simulink model "Main_Simulink"  (R2023b)
settings: Solver=FixedStepDiscrete  StartTime=0.0  StopTime=inf  FixedStep=0.001  RelTol=1e-3
undefined symbols (not defined in the file or in its folder): battery_builder_rtmsupport, gcbh, Initial_SOC
libraries: nesl_utility x118, pack_105s34p_structured_lib x105, fl_lib x14, ee_lib x7, dspstat3 x6, BatteryBalancing x1, deeplib x1
(part 3 of 10)

== system Main_Simulink/Battery Management System/State of Power Estimation System/Maximum Charge Power Limits/For Each Subsystem1 ==
  Temp : Inport  Partition=on  PartitionDimension=1  PartitionWidth=1  PartitionOffset=0
  HVBatSOCMin : Inport  Port=2
  For Each : ForEach  DisableCoverage=on
  Pack Charge Power Limit - 10s : Lookup_n-D  BreakpointsForDimension1=[-30;-20;-10;0;10;20;30;40;50;60]  BreakpointsForDimension2=[0 5 10 15 20 25 30 35 40 45 50 55 60 65 70 75 80 85 90 95 100]  Table=[0 0 0 0 0 0 0 0 0 0 0 0 0 0 0 0 0 0 0 0 0;0 0 0 0 0 0 0 0 0 0 0 0 0 0 0 0 0 0 0 0 0;19.76749 19.76749 19.65082 20.01926 20.36403 19.91161 19.53766 17.74126 15.90855 13.98243 12.04796 10.11331 8.150748 6.165785 4.146483 4.194749 4.24254 2.863269 1.449165 0.729806 0;37.15349 37.25908 37.36467 37.99491 38.68739 37.01292 35.57943 34.03129 32.33249 28.38431 24.39997 22.5555 20.67389 16.66823 12.60507 10.58905 8.539529 6.477517 4.366351 2.192535 0;50.75138 51.59179 51.65872 52.84392 54.27789 52.74104 51.43037 49.99522 48.55512 44.79444 41.00328 35.11689 29.12726 25.2468 21.25129 17.16492 12.9983 10.91332 8.795933 4.432558 0;67.50776 69.05614 69.22503 70.87652 72.7677 72.79337 73.0761 69.11144 65.03528 61.39678 57.74562 50.54301 43.23853 38.08701 32.7453 27.30376 21.75319 18.2489 14.69784 7.398185 0;75.51099 77.37549 77.95205 79.80169 81.84837 82.63384 83.74967 78.51018 73.16383 69.64374 66.0563 58.24337 50.28199 44.49695 38.47487 32.35472 26.12019 21.90894 17.64118 8.874131 0;74.46151 76.49357 77.35464 79.22241 81.36253 82.08661 83.22665 78.09122 72.77178 69.28399 65.77915 57.99753 50.09838 44.31755 38.34415 32.22712 26.01267 21.84759 17.61682 8.847446 0;48.00354 49.35825 50.19251 51.64039 53.2093 53.79276 54.56109 51.26258 47.84552 45.59639 43.32059 38.26118 33.1039 29.30947 25.39243 21.36695 17.26419 14.51359 11.71338 5.890391 0;0 0 0 0 0 0 0 0 0 0 0 0 0 0 0 0 0 0 0 0 0]  InternalRulePriority=Speed  RndMeth=Simplest
      settings: InputPortMap=u0,u1
  Out1 : Outport  ConcatenationDimension=1
  wires:
  HVBatSOCMin/1 -> Pack Charge Power Limit - 10s/2
  Temp/1 -> Pack Charge Power Limit - 10s/1
  Pack Charge Power Limit - 10s/1 -> Out1/1

== system Main_Simulink/Battery Management System/State of Power Estimation System/Maximum Charge Power Limits/For Each Subsystem2 ==
  Temp : Inport  Partition=on  PartitionDimension=1  PartitionWidth=1  PartitionOffset=0
  HVBatSOCMin : Inport  Port=2
  For Each : ForEach  DisableCoverage=on
  Pack Charge Power Limit - 2s : Lookup_n-D  BreakpointsForDimension1=[-30;-20;-10;0;10;20;30;40;50;60]  BreakpointsForDimension2=[0 5 10 15 20 25 30 35 40 45 50 55 60 65 70 75 80 85 90 95 100]  Table=[0 0 0 0 0 0 0 0 0 0 0 0 0 0 0 0 0 0 0 0 0;0 0 0 0 0 0 0 0 0 0 0 0 0 0 0 0 0 0 0 0 0;19.58352 19.58352 19.45651 19.84169 20.21864 19.8213 19.46671 17.67557 15.85694 13.94558 12.01771 10.09422 8.137316 6.159089 4.143376 4.191016 4.238837 2.861684 1.448811 0.72974 0;36.49456 36.60015 36.70574 37.48533 38.32484 36.81065 35.41273 33.83658 32.2081 28.27762 24.32648 22.49047 20.61798 16.63012 12.57878 10.57114 8.529705 6.471868 4.364553 2.192111 0;49.59029 50.43071 50.70087 52.14778 53.75303 52.35297 51.03415 49.65909 48.22489 44.53214 40.77991 34.95857 29.0243 25.154 21.18801 17.12293 12.9785 10.89967 8.788762 4.430448 0;65.59661 67.14499 67.90263 69.84698 72.06978 72.21885 72.5005 68.58984 64.57818 61.01484 57.37573 50.30478 43.06975 37.92462 32.63123 27.2283 21.70777 18.22059 14.68121 7.393929 0;73.18842 75.05293 76.34885 78.58837 81.05583 82.06849 83.18148 77.97854 72.71563 69.2522 65.72517 57.97825 50.09367 44.30032 38.34697 32.26844 26.06097 21.87292 17.6235 8.869533 0;71.97071 74.00277 75.69889 78.01635 80.51607 81.53568 82.69007 77.60201 72.42077 68.96612 65.46512 57.75822 49.92863 44.16534 38.24005 32.15085 25.96253 21.81627 17.60159 8.843684 0;46.89652 48.25122 49.45662 51.10436 52.8331 53.5479 54.32261 51.04516 47.68952 45.45511 43.18102 38.15483 33.02845 29.24182 25.34616 21.33306 17.24191 14.49967 11.70661 5.888719 0;0 0 0 0 0 0 0 0 0 0 0 0 0 0 0 0 0 0 0 0 0]  InternalRulePriority=Speed  RndMeth=Simplest
      settings: InputPortMap=u0,u1
  Out1 : Outport  ConcatenationDimension=1
  wires:
  HVBatSOCMin/1 -> Pack Charge Power Limit - 2s/2
  Temp/1 -> Pack Charge Power Limit - 2s/1
  Pack Charge Power Limit - 2s/1 -> Out1/1

== system Main_Simulink/Battery Management System/State of Power Estimation System/Maximum Charge Power Limits/For Each Subsystem3 ==
  Temp : Inport  Partition=on  PartitionDimension=1  PartitionWidth=1  PartitionOffset=0
  HVBatSOCMin : Inport  Port=2
  For Each : ForEach  DisableCoverage=on
  Pack Charge Power Limit - 30s : Lookup_n-D  BreakpointsForDimension1=[-30;-20;-10;0;10;20;30;40;50;60]  BreakpointsForDimension2=[0 5 10 15 20 25 30 35 40 45 50 55 60 65 70 75 80 85 90 95 100]  Table=[0 0 0 0 0 0 0 0 0 0 0 0 0 0 0 0 0 0 0 0 0;0 0 0 0 0 0 0 0 0 0 0 0 0 0 0 0 0 0 0 0 0;0 0 0 0 0 0 0 0 0 0 0 0 0 0 0 0 0 0 0 0 0;8.039485 8.064123 8.088761 8.279835 8.501733 8.660965 8.837547 8.974482 9.110076 7.866004 6.603531 6.683109 6.761689 5.473014 4.152702 4.200954 4.248799 2.866871 1.450526 0.729607 0;11.3011 11.5012 11.63529 12.01056 12.40712 12.57062 12.75608 12.93391 13.1115 13.24873 13.3883 13.56159 13.73198 13.9362 14.11972 13.57803 13.02453 10.92908 8.805357 4.435029 0;14.96331 15.33197 15.57367 16.06785 16.58759 16.79556 17.03852 17.27949 17.51753 17.70142 17.88948 18.11963 18.34425 18.62175 18.85959 18.86453 18.86253 15.32536 11.7483 5.916568 0;20.71779 21.26037 21.60042 22.24946 22.91092 23.18255 23.52677 23.84754 24.16825 24.42631 24.69339 25.006 25.31353 24.50762 23.60729 22.69796 21.75837 17.50956 13.21299 6.651374 0;28.3715 29.17787 29.59744 30.45927 31.35956 31.68052 32.17173 32.61593 33.0527 33.41197 33.7704 34.18493 34.60144 31.54245 28.32199 25.02635 21.66624 17.46263 13.19626 6.631388 0;16.60354 17.08736 17.43194 18.00695 18.5958 18.82348 19.11245 19.38268 19.65023 19.86546 20.08039 20.33233 20.58498 20.88514 21.15023 17.79983 14.38194 13.06513 11.72123 5.892346 0;0 0 0 0 0 0 0 0 0 0 0 0 0 0 0 0 0 0 0 0 0]  InternalRulePriority=Speed  RndMeth=Simplest
      settings: InputPortMap=u0,u1
  Out1 : Outport  ConcatenationDimension=1
  wires:
  HVBatSOCMin/1 -> Pack Charge Power Limit - 30s/2
  Temp/1 -> Pack Charge Power Limit - 30s/1
  Pack Charge Power Limit - 30s/1 -> Out1/1

== system Main_Simulink/Battery Management System/State of Power Estimation System/Maximum Charge Power Limits/For Each Subsystem4 ==
  Temp : Inport  Partition=on  PartitionDimension=1  PartitionWidth=1  PartitionOffset=0
  HVBatSOCMin : Inport  Port=2
  For Each : ForEach  DisableCoverage=on
  Pack Charge Power Limit - 180s : Lookup_n-D  BreakpointsForDimension1=[-30;-20;-10;0;10;20;30;40;50;60]  BreakpointsForDimension2=[0 5 10 15 20 25 30 35 40 45 50 55 60 65 70 75 80 85 90 95 100]  Table=[0 0 0 0 0 0 0 0 0 0 0 0 0 0 0 0 0 0 0 0 0;0 0 0 0 0 0 0 0 0 0 0 0 0 0 0 0 0 0 0 0 0;0 0 0 0 0 0 0 0 0 0 0 0 0 0 0 0 0 0 0 0 0;8.200519 8.225157 8.249795 8.449791 8.628751 8.713708 8.900788 9.041006 9.17303 7.90902 6.631868 6.710427 6.788544 5.492872 4.164691 4.209532 4.257341 2.870725 1.451275 0.729786 0;11.73069 11.93079 11.98528 12.24386 12.50444 12.65479 12.85775 13.02347 13.18717 13.32159 13.46314 13.63484 13.8141 14.0262 14.18781 13.64706 13.09032 10.96258 8.823694 4.44097 0;15.75103 16.11969 16.16875 16.4414 16.72958 16.92433 17.19946 17.41833 17.62262 17.80263 17.99554 18.22015 18.4672 18.74861 18.95158 18.96809 18.96715 15.37262 11.77152 5.926242 0;22.12594 22.66852 22.66387 22.907 23.15513 23.4058 23.7974 24.09552 24.35036 24.60225 24.8676 25.17956 25.53041 24.68474 23.72629 22.82709 21.87994 17.56221 13.23562 6.661459 0;31.06494 31.87131 31.6124 31.82007 31.86082 32.06269 32.65549 33.0561 33.38556 33.68284 34.05866 34.47747 34.96167 31.81577 28.4752 25.16758 21.7805 17.51312 13.21427 6.63946 0;17.57318 18.057 18.15732 18.49684 18.77626 18.96106 19.2866 19.54114 19.77006 19.96297 20.18416 20.43764 20.71466 21.00661 21.23642 17.87188 14.43273 13.09353 11.73546 5.898724 0;0 0 0 0 0 0 0 0 0 0 0 0 0 0 0 0 0 0 0 0 0]  InternalRulePriority=Speed  RndMeth=Simplest
      settings: InputPortMap=u0,u1
  Out1 : Outport  ConcatenationDimension=1
  wires:
  HVBatSOCMin/1 -> Pack Charge Power Limit - 180s/2
  Temp/1 -> Pack Charge Power Limit - 180s/1
  Pack Charge Power Limit - 180s/1 -> Out1/1

== system Main_Simulink/Battery Management System/State of Power Estimation System/Maximum Discharge Power Limits/For Each Subsystem ==
  Temp : Inport  Partition=on  PartitionDimension=1  PartitionWidth=1  PartitionOffset=0
  HVBatSOCMin : Inport  Port=2
  For Each : ForEach  DisableCoverage=on
  Pack Discharge Power Limit - 2s : Lookup_n-D  BreakpointsForDimension1=[-30;-20;-10;0;10;20;30;40;50;60]  BreakpointsForDimension2=[0 5 10 15 20 25 30 35 40 45 50 55 60 65 70 75 80 85 90 95 100]  Table=[0 0 0 0 0 0 0 0 0 0 0 0 0 0 0 0 0 0 0 0 0;0 1.6 3.2 6.9 10.5 10.9 11.4 11.6 11.8 12 12.2 18 23.6 24 24.4 24.8 25.1 25.5 25.9 26.4 26.8;0 2.8 5.4 8.4 11.5 22.7 33.8 34.4 35 35.5 35.9 41.8 47.8 48.5 49.2 49.9 50.5 51.4 52.3 58.6 65.1;0 5.4 10.7 21.7 33 39.3 45.5 46.4 47.2 53.2 59.1 59.9 60.8 67.2 73.8 74.7 75.6 76.8 78.1 78.7 79.6;0 10.9 21.9 33.9 46.6 53 59.5 66.1 73 73.8 74.6 81.6 88.7 90 91.2 98.6 106.4 113.2 120.4 121.6 122.7;0 16.2 32.8 50.5 69.1 75.8 82.6 89.5 96.7 97.8 98.9 106.2 113.5 115.2 116.7 124.5 132.3 139.8 147.3 148.9 150.4;0 16.3 33.1 97.7 160.7 163.9 166.7 169.9 172.6 175 177.1 179.7 182.2 185.1 187.7 190.3 192.9 195.2 197.2 199.5 201.3;0 16.2 33 97.8 162.1 164.9 168.1 170.8 173.9 176.1 178.2 180.7 183.2 185.7 188.4 191 194.5 196.2 198.7 200.6 202.2;0 10.9 22.2 34.3 47.2 53.8 60.5 67.3 74.3 75.2 76 83.2 90.5 91.7 93 94.2 95.6 103.1 110.9 111.9 112.8;0 0 0 0 0 0 0 0 0 0 0 0 0 0 0 0 0 0 0 0 0]  InternalRulePriority=Speed  RndMeth=Simplest
      settings: InputPortMap=u0,u1
  Out1 : Outport  ConcatenationDimension=1
  wires:
  HVBatSOCMin/1 -> Pack Discharge Power Limit - 2s/2
  Temp/1 -> Pack Discharge Power Limit - 2s/1
  Pack Discharge Power Limit - 2s/1 -> Out1/1

== system Main_Simulink/Battery Management System/State of Power Estimation System/Maximum Discharge Power Limits/For Each Subsystem1 ==
  Temp : Inport  Partition=on  PartitionDimension=1  PartitionWidth=1  PartitionOffset=0
  HVBatSOCMin : Inport  Port=2
  For Each : ForEach  DisableCoverage=on
  Pack Discharge Power Limit - 10s : Lookup_n-D  BreakpointsForDimension1=[-30;-20;-10;0;10;20;30;40;50;60]  BreakpointsForDimension2=[0 5 10 15 20 25 30 35 40 45 50 55 60 65 70 75 80 85 90 95 100]  Table=[0 0 0 0 0 0 0 0 0 0 0 0 0 0 0 0 0 0 0 0 0;0 1.6 3.2 6.8 10.4 10.9 11.3 11.6 11.8 12 12.1 17.9 23.4 23.8 24.2 24.6 24.9 25.3 25.8 26.2 26.6;0 2.7 5.4 8.3 11.4 22.6 33.5 34.2 34.8 35.2 35.6 41.4 47.2 48 48.7 49.4 50 50.8 51.7 57.9 64;0 5.4 10.6 21.4 32.7 39 45.2 46.1 47 52.9 58.7 59.5 60.2 66.6 73 73.8 74.6 75.8 77.1 78 78.7;0 10.8 21.7 33.6 46.1 52.5 58.9 65.4 72.1 73 73.8 80.6 87.6 88.8 90 97 104.3 111.3 118.4 119.7 120.3;0 16.1 32.4 50 68.4 75 81.7 83.1 84.5 91.1 97.8 105 112.1 113.6 115.1 122.5 130.1 137.7 145.1 146.8 147.6;0 16.2 32.8 61 90.2 97.2 104.2 111.2 118.5 125.4 132.3 139.7 147.2 154.9 162.3 170.2 178 186.2 194.3 196.5 197.2;0 16.1 32.7 61 90.4 97.4 104.5 111.8 119.1 126 133.1 140.3 148 155.4 163.2 171.2 179.5 187.6 196.5 198.3 198.8;0 10.8 22.1 34.1 46.9 53.5 60.2 67 73.9 74.7 75.6 82.6 89.9 91 92.3 93.5 94.8 102.4 110.3 111.2 111.8;0 0 0 0 0 0 0 0 0 0 0 0 0 0 0 0 0 0 0 0 0]  InternalRulePriority=Speed  RndMeth=Simplest
      settings: InputPortMap=u0,u1
  Out1 : Outport  ConcatenationDimension=1
  wires:
  HVBatSOCMin/1 -> Pack Discharge Power Limit - 10s/2
  Temp/1 -> Pack Discharge Power Limit - 10s/1
  Pack Discharge Power Limit - 10s/1 -> Out1/1

== system Main_Simulink/Battery Management System/State of Power Estimation System/Maximum Discharge Power Limits/For Each Subsystem2 ==
  Temp : Inport  Partition=on  PartitionDimension=1  PartitionWidth=1  PartitionOffset=0
  HVBatSOCMin : Inport  Port=2
  For Each : ForEach  DisableCoverage=on
  Pack Discharge Power Limit - 30s : Lookup_n-D  BreakpointsForDimension1=[-30;-20;-10;0;10;20;30;40;50;60]  BreakpointsForDimension2=[0 5 10 15 20 25 30 35 40 45 50 55 60 65 70 75 80 85 90 95 100]  Table=[0 0 0 0 0 0 0 0 0 0 0 0 0 0 0 0 0 0 0 0 0;0 1.6 3.2 6.7 10.2 10.7 11.2 11.5 11.7 11.9 12 17.7 23.1 23.5 24 24.3 24.7 25.1 25.5 25.9 26.3;0 2.7 5.3 8.3 11.3 22.4 33 33.7 34.4 34.8 35.2 40.8 46.4 47.2 47.9 48.6 49.2 49.9 50.8 56.9 62.8;0 5.4 10.5 21 32.2 38.5 44.7 45.5 46.5 52.2 57.9 58.6 59.4 65.5 71.7 72.3 73.1 74.3 75.7 76.7 77.4;0 10.7 21.3 33.1 45.5 51.8 58.2 64.6 71.1 71.9 72.8 79.3 86.1 87.3 88.2 94.8 101.8 108.9 116 117.3 117.4;0 14.1 28.5 44 60.3 70.5 80.5 87.2 94.1 95.2 96.3 103.3 110.2 111.4 112.7 119.9 127.1 138.5 150.1 152 151.7;0 16 32.3 49.6 67.9 80.1 92 98.9 106 107.3 108.6 115.7 123 124.2 125.9 133.2 140.8 154.3 168.5 170.5 170;0 15.9 32.2 49.5 68 80.2 92.4 99.4 106.6 107.9 109.1 116.3 123.6 124.8 126.6 134.1 141.8 155.5 170.5 172.4 171.8;0 10.7 21.8 33.8 46.5 53 59.6 66.3 73.2 74.1 74.9 81.9 89 90 91.3 92.5 93.7 101.3 109.4 110.5 110.6;0 0 0 0 0 0 0 0 0 0 0 0 0 0 0 0 0 0 0 0 0]  InternalRulePriority=Speed  RndMeth=Simplest
      settings: InputPortMap=u0,u1
  Out1 : Outport  ConcatenationDimension=1
  wires:
  HVBatSOCMin/1 -> Pack Discharge Power Limit - 30s/2
  Temp/1 -> Pack Discharge Power Limit - 30s/1
  Pack Discharge Power Limit - 30s/1 -> Out1/1

== system Main_Simulink/Battery Management System/State of Power Estimation System/Maximum Discharge Power Limits/For Each Subsystem3 ==
  Temp : Inport  Partition=on  PartitionDimension=1  PartitionWidth=1  PartitionOffset=0
  HVBatSOCMin : Inport  Port=2
  For Each : ForEach  DisableCoverage=on
  Pack Discharge Power Limit - 180s : Lookup_n-D  BreakpointsForDimension1=[-30;-20;-10;0;10;20;30;40;50;60]  BreakpointsForDimension2=[0 5 10 15 20 25 30 35 40 45 50 55 60 65 70 75 80 85 90 95 100]  Table=[0 0 0 0 0 0 0 0 0 0 0 0 0 0 0 0 0 0 0 0 0;0 1.1 2.1 3.6 5.2 5.5 5.7 5.9 6 6.1 6.2 12 17.4 17.7 18 18.3 18.6 18.9 19.2 19.5 19.9;0 1.6 3.1 4.4 5.7 14.1 22.3 22.7 23.1 28.5 33.7 34.1 34.6 35.2 35.9 36.4 36.8 37.2 37.9 38.6 39;0 4.6 8.5 14.2 20.9 27.2 33.4 34 34.7 40.3 45.7 46.3 46.9 52.8 58.3 58.7 59.4 60.2 61.6 63.2 63.7;0 7.5 15.2 23.9 33.2 39.8 45.8 51.8 57.9 58.6 59.3 65.6 72.1 72.8 73.1 78.9 84.8 92 100.3 101.4 99.1;0 9.3 18.9 26 33.8 51 67.1 73.3 79.6 80.7 81.7 91.8 102 102.1 102.3 105.1 108 113.2 119.2 120.5 117.1;0 9 18.3 23.7 29.9 50.4 69.7 75.3 80.9 82.1 83.1 94.4 105.8 105.6 106.5 107.8 109.2 112.4 116.1 117.3 114.5;0 6.3 12.9 16.7 21 37.1 52.6 56.3 60.1 60.8 61.5 71.2 81 81.2 82.2 82.9 84.3 86.1 88.6 89.5 88.5;0 2.7 5.5 19.3 33.9 35.4 35.9 36.5 37.1 37.6 38 38.6 39.1 39.5 40 40.4 41 41.6 42.4 42.8 42.8;0 0 0 0 0 0 0 0 0 0 0 0 0 0 0 0 0 0 0 0 0]  InternalRulePriority=Speed  RndMeth=Simplest
      settings: InputPortMap=u0,u1
  Out1 : Outport  ConcatenationDimension=1
  wires:
  HVBatSOCMin/1 -> Pack Discharge Power Limit - 180s/2
  Temp/1 -> Pack Discharge Power Limit - 180s/1
  Pack Discharge Power Limit - 180s/1 -> Out1/1
